simulink model "lin_flapping_mdl"  (Simulink 7.7)
settings: Solver=ode45  StartTime=0.0  StopTime=5  RelTol=1e-3
settings Model: Creator=Administrator  LastModifiedBy=Administrator
settings DataIOCC: LimitDataPoints=off

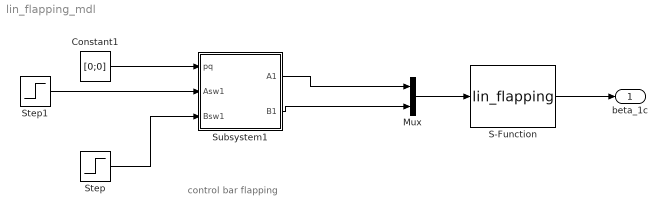
== system lin_flapping_mdl ==
  note: control bar flapping
  Constant1 : Constant  Value=[0;0]
  Mux : Mux  Inputs=2
  S-Function : S-Function  RequirementInfo={} %GIDa_6ad0541c_1708_4cdf_8ca9_8fc84baf1198  FunctionName=lin_flapping  EnableBusSupport=off
  Step : Step  Time=0.2  After=0  SampleTime=0
  Step1 : Step  Time=0.2  SampleTime=0
  Subsystem1 : Subsystem  mask{Ksw=0.2, Kcr=0.8}
  beta_1c : Outport
  wires:
  Mux/1 -> S-Function/1
  Subsystem1/1(A1) -> Mux/1
  Subsystem1/2(B1) -> Mux/2
  S-Function/1 -> beta_1c/1
  Step/1 -> Subsystem1/3(Bsw1)
  Step1/1 -> Subsystem1/2(Asw1)
  Constant1/1 -> Subsystem1/1(pq)

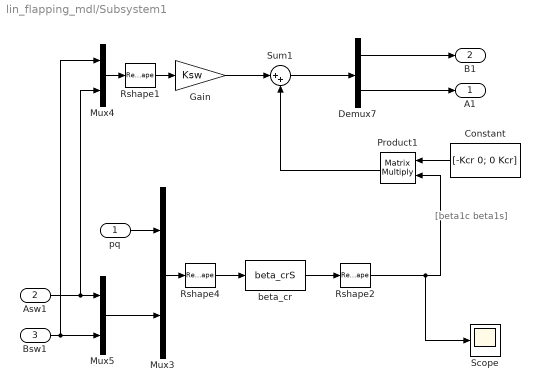
== system lin_flapping_mdl/Subsystem1 ==
  note: [beta1c
      | beta1s]
  pq : Inport
  Asw1 : Inport  Port=2
  Bsw1 : Inport  Port=3
  Constant : Constant  Value=[-Kcr 0; 0 Kcr]
  Demux7 : Demux  Outputs=[1 1]
  Gain : Gain  Gain=Ksw
  Mux3 : Mux  Inputs=2
  Mux4 : Mux  Inputs=2
  Mux5 : Mux  Inputs=2
  Product1 : Product  Multiplication=Matrix(*)  RndMeth=Zero
  Rshape1 : Reshape  OutputDimensionality=Column vector (2-D)
  Rshape2 : Reshape  OutputDimensionality=Column vector (2-D)
  Rshape4 : Reshape  OutputDimensionality=Column vector (2-D)
  Scope : Scope
      settings: YMin=-1  YMax=2
  Sum1 : Sum  Inputs=|++
  beta_cr : S-Function  FunctionName=beta_crS  EnableBusSupport=off
  A1 : Outport
  B1 : Outport  Port=2
  wires:
  Rshape4/1 -> beta_cr/1
  Mux3/1 -> Rshape4/1
  Product1/1 -> Sum1/2
  Mux4/1 -> Rshape1/1
  Rshape1/1 -> Gain/1
  Sum1/1 -> Demux7/1
  Gain/1 -> Sum1/1
  Constant/1 -> Product1/1
  Bsw1/1 -> Mux5/2, Mux4/1
  Asw1/1 -> Mux5/1, Mux4/2
  Demux7/1 -> B1/1
  Demux7/2 -> A1/1
  beta_cr/1 -> Rshape2/1
  Rshape2/1 -> Product1/2, Scope/1
  Mux5/1 -> Mux3/2
  pq/1 -> Mux3/1
